simulink model "ME430MidtermSimulink"  (R2020b)
settings: Solver=VariableStepAuto  StartTime=0.0  StopTime=500  RelTol=1e-3
undefined symbols (not defined in the file or in its folder): Input
libraries: simulink x2
settings Model: Creator=jaagt  LastModifiedBy=jaagt

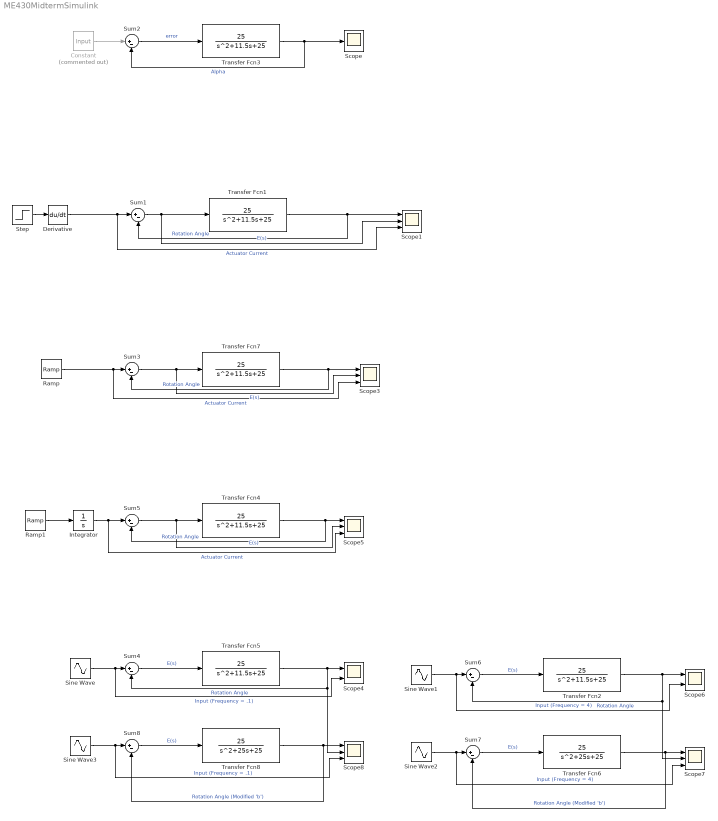
== system ME430MidtermSimulink ==
  Constant : Constant  Commented=on  Value=Input
  Derivative : Derivative
  Integrator : Integrator
  Ramp : simulink/Sources/Ramp  slope=1  start=0  InitialOutput=0
  Ramp1 : simulink/Sources/Ramp  slope=1  start=0  InitialOutput=0
  Scope : Scope
  Scope{1,3,5,7..8} (5 alike) : Scope  NumInputPorts=3
  Scope4 : Scope  NumInputPorts=2
  Scope6 : Scope  NumInputPorts=2
  Sine Wave : Sin  Frequency=.1  SampleTime=0
  Sine Wave1 : Sin  Frequency=4  SampleTime=0
  Sine Wave2 : Sin  Frequency=4  SampleTime=0
  Sine Wave3 : Sin  Frequency=.1  SampleTime=0
  Step : Step  Time=.01  SampleTime=0
  Sum{1..8} (8 alike) : Sum  Inputs=|+-
  Transfer Fcn{1..5,7} (6 alike) : TransferFcn  Numerator=25  Denominator=[1 11.5 25]
  Transfer Fcn6 : TransferFcn  Numerator=25  Denominator=[1 25 25]
  Transfer Fcn8 : TransferFcn  Numerator=25  Denominator=[1 25 25]
  wires:
  Ramp1/1 -> Integrator/1
  Integrator/1 -> Scope5/3, Sum5/1  "Actuator Current"
  Sum5/1 -> Transfer Fcn4/1, Scope5/2  "E(s)"
  Transfer Fcn5/1 -> Scope8/2, Sum4/2, Scope4/1  "Rotation Angle"
  Sum3/1 -> Transfer Fcn7/1, Scope3/2  "E(s)"
  Sum4/1 -> Transfer Fcn5/1  "E(s)"
  Transfer Fcn4/1 -> Sum5/2, Scope5/1  "Rotation Angle"
  Ramp/1 -> Scope3/3, Sum3/1  "Actuator Current"
  Sum2/1 -> Transfer Fcn3/1  "error"
  Sum1/1 -> Scope1/2, Transfer Fcn1/1  "E(s)"
  Sine Wave/1 -> Scope4/2, Sum4/1  "Input (Frequency = .1)"
  Derivative/1 -> Scope1/3, Sum1/1  "Actuator Current"
  Constant/1 -> Sum2/1
  Transfer Fcn3/1 -> Scope/1, Sum2/2  "Alpha"
  Transfer Fcn7/1 -> Sum3/2, Scope3/1  "Rotation Angle"
  Transfer Fcn1/1 -> Sum1/2, Scope1/1  "Rotation Angle"
  Step/1 -> Derivative/1
  Sine Wave1/1 -> Scope6/2, Sum6/1  "Input (Frequency = 4)"
  Sum6/1 -> Transfer Fcn2/1  "E(s)"
  Transfer Fcn2/1 -> Scope7/2, Sum6/2, Scope6/1  "Rotation Angle"
  Sum7/1 -> Transfer Fcn6/1  "E(s)"
  Transfer Fcn6/1 -> Sum7/2, Scope7/1  "Rotation Angle (Modified 'b')"
  Sine Wave2/1 -> Scope7/3, Sum7/1  "Input (Frequency = 4)"
  Sine Wave3/1 -> Scope8/3, Sum8/1  "Input (Frequency = .1)"
  Sum8/1 -> Transfer Fcn8/1  "E(s)"
  Transfer Fcn8/1 -> Sum8/2, Scope8/1  "Rotation Angle (Modified 'b')"
